simulink model "mecanical_model_simulink"  (R2023a)
settings: Solver=VariableStepAuto  StartTime=0.0  StopTime=50  RelTol=1e-3
values from neighbouring files (symbols this model uses):
  dem = [taux 1]    [servo_simulation.m]
settings Model: Creator=IDEAL SOFT  LastModifiedBy=IDEAL SOFT
settings RTWCC: GenCodeOnly=on

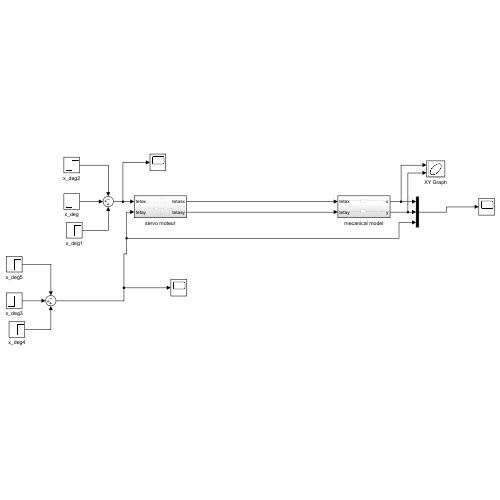
[thumbnail: Simulink's stored preview of the top-level diagram]
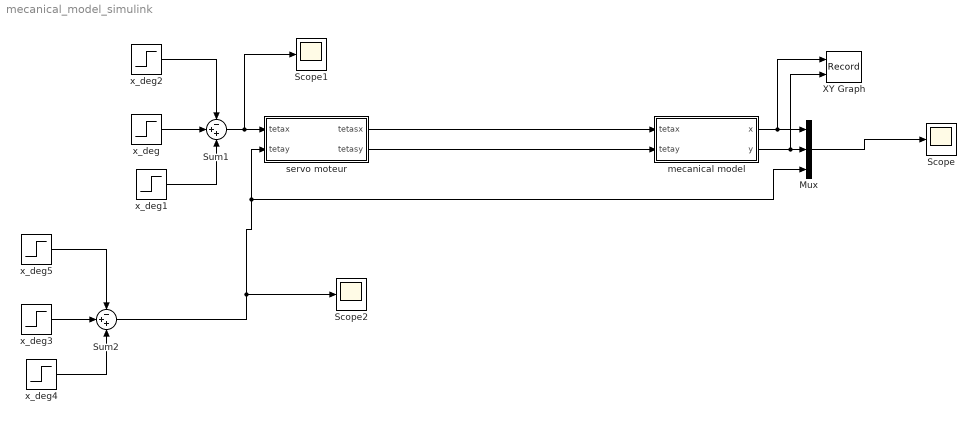
== system mecanical_model_simulink ==
  Mux : Mux  Inputs=3
  Scope : Scope
  Scope1 : Scope
  Scope2 : Scope
  Sum1 : Sum  Inputs=-++
  Sum2 : Sum  Inputs=-++
  XY Graph : Record  RecordToWorkspace=on  FileSettingsInternal="{\"entries\":[{\"content\":{\"excelSettings\":{\"content\":{},\"type\":\"Streamout.ExcelSettings\"}},\"type\":\"Streamout.FileSettingStorage\",\"uuid\":\"0d7345cf-e264-44ac-8379-3d4de4675625\"}],\"packageUris\":[\"http://schema.mathworks.com/mf0/streamout_blocks/R2020a\"],\"version\":\"1.0\"}"  Layout=[1 1]  SignalsInternal="{\"entries\":[{\"content\":{\"signals\":[{\"content\":{\"blockPath\":[\"mecanical_model_simulink/XY Graph\"],\"dimensions\":[1],\"domain\":\"mecanical_model_simulink/XY Graph\",\"lineColor\":\"#a2142f\",\"plots\":[1],\"port\":1,\"sid\":[\"\"],\"signalID\":593,\"signalName\":\"mecanical model:1\"},\"type\":\"RecordBlkView.Signal\",\"uuid\":\"3c06d480-1d2e-4741-930e-6bac143f6451\"},{\"content\":{\"blockPath\":[\"mecanical_model_simulink/XY Graph\"],\"dimensions\":[1],\"domain\":\"mecanical_model_simulink/XY Graph\",\"lineColor\":\"#139fff\",\"plots\":[1],\"port\":2,\"sid\":[\"\"],\"signalID\":597,\"signalName\":\"mecanical model:2\"},\"type\":\"RecordBlkView.Signal\",\"uuid\":\"8a5b9cd0-4292-4105-9623-7b500a0137e2\"}]},\"type\":\"RecordBlkView.InputSignals\",\"uuid\":\"b5083803-8b0a-4987-b666-7a16f106ea54\"}],\"packageUris\":[\"http://schema.mathworks.com/mf0/streamout_blocks/R2020a\"],\"version\":\"1.0\"}"  VisualizationBindings="{\"xyplotplugin\":{\"info\":[{\"series\":[{\"bindingParametersList\":[{\"parameter\":\"X-Axis\",\"signalID\":593,\"signalName\":\"mecanical model:1\"},{\"parameter\":\"Y-Axis\",\"signalID\":597,\"signalName\":\"mecanical model:2\"}],\"seriesID\":17123}],\"subplotID\":1}]}}"  CompatibilityTag=XY
  mecanical model : Subsystem
  servo moteur : Subsystem
  x_deg : Step  Time=10  After=5  SampleTime=0
  x_deg1 : Step  Time=30  After=5  SampleTime=0
  x_deg2 : Step  Time=20  After=10  SampleTime=0
  x_deg3 : Step  Time=10  After=5  SampleTime=0
  x_deg4 : Step  Time=30  After=5  SampleTime=0
  x_deg5 : Step  Time=20  After=10  SampleTime=0
  wires:
  servo moteur/1(tetasx) -> mecanical model/1(tetax)
  servo moteur/2(tetasy) -> mecanical model/2(tetay)
  Mux/1 -> Scope/1
  mecanical model/2(y) -> XY Graph/2, Mux/2
  mecanical model/1(x) -> XY Graph/1, Mux/1
  Sum2/1 -> Mux/3, servo moteur/2(tetay), Scope2/1
  x_deg2/1 -> Sum1/1
  x_deg/1 -> Sum1/2
  Sum1/1 -> Scope1/1, servo moteur/1(tetax)
  x_deg1/1 -> Sum1/3
  x_deg3/1 -> Sum2/2
  x_deg4/1 -> Sum2/3
  x_deg5/1 -> Sum2/1

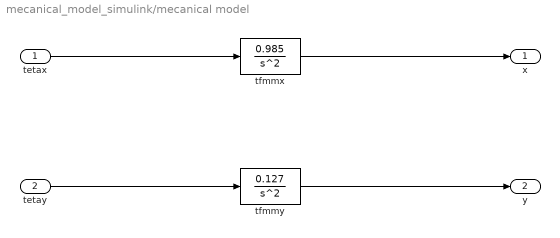
== system mecanical_model_simulink/mecanical model ==
  tetax : Inport
  tetay : Inport  Port=2
  tfmmx : TransferFcn  Numerator=0.985  Denominator=[1 0 0]
  tfmmy : TransferFcn  Numerator=0.127  Denominator=[1 0 0]
  x : Outport
  y : Outport  Port=2
  wires:
  tetax/1 -> tfmmx/1
  tfmmx/1 -> x/1
  tetay/1 -> tfmmy/1
  tfmmy/1 -> y/1

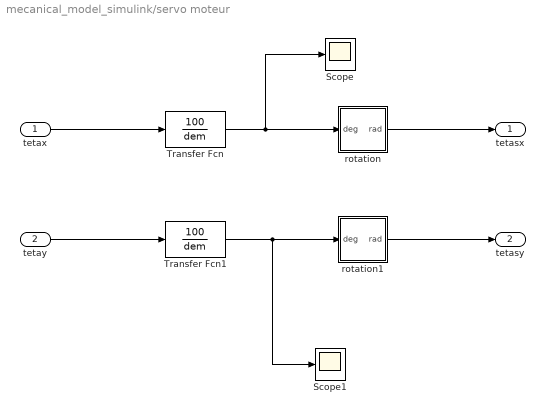
== system mecanical_model_simulink/servo moteur ==
  tetax : Inport
  tetay : Inport  Port=2
  Scope : Scope
  Scope1 : Scope
  Transfer Fcn : TransferFcn  Numerator=100  Denominator=dem
  Transfer Fcn1 : TransferFcn  Numerator=100  Denominator=dem
  rotation : Subsystem
  rotation1 : Subsystem
  tetasx : Outport
  tetasy : Outport  Port=2
  wires:
  tetax/1 -> Transfer Fcn/1
  tetay/1 -> Transfer Fcn1/1
  Transfer Fcn/1 -> Scope/1, rotation/1(deg)
  rotation/1(rad) -> tetasx/1
  Transfer Fcn1/1 -> Scope1/1, rotation1/1(deg)
  rotation1/1(rad) -> tetasy/1

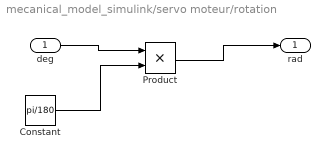
== system mecanical_model_simulink/servo moteur/rotation ==
  deg : Inport
  Constant : Constant  Value=pi/180
  Product : Product
  rad : Outport
  wires:
  deg/1 -> Product/1
  Product/1 -> rad/1
  Constant/1 -> Product/2

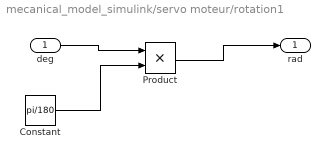
== system mecanical_model_simulink/servo moteur/rotation1 ==
  deg : Inport
  Constant : Constant  Value=pi/180
  Product : Product
  rad : Outport
  wires:
  deg/1 -> Product/1
  Product/1 -> rad/1
  Constant/1 -> Product/2
